simulink model "cooling_v3"  (R2022b)
settings: Solver=FixedStepDiscrete  StartTime=0.0  StopTime=10.0  FixedStep=0.005  RelTol=1e-3  EnableMultiTasking=on
PreLoadFcn:
  | try, model_open; catch, disp('Error occurred while executing model pre-load callback: model_open.m'); disp('Please assure that the MATLAB working directory is set to the model directory before opening.'); end
InitFcn:
  | try, model_open; catch, end
undefined symbols (not defined in the file): GCM, raptor_get_safe_string, raptor_xcp_function, sigbuilder_block
libraries: Raptor_lib x39, simulink x8, simulink_extras x1, dspswit3 x1, dspstat3 x1
CloseFcn:
  | try, model_close; catch, end
settings Model: Raptor_Target=GCM-1793-196-1503  Raptor_Calloc=NonVolatile (EEPROM)  RaptorUIDSize=4  RaptorBuildNum=0  Raptor_ecuaddr=11  RaptorFaultManager=Standard  RaptorFaultManagerAddXYCounts=1  Raptor_IsLiteMode=0  Creator=Ben  LastModifiedBy=jackh
settings SolverCC: AlgebraicLoopSolver=TrustRegion
settings DataIOCC: LimitDataPoints=on  SaveFormat=Array  SignalLoggingSaveFormat=ModelDataLogs  ReturnWorkspaceOutputs=off
settings OptimizationCC: DefaultParameterBehavior=Inlined  ExpressionDepthLimit=2147483647  InitFltsAndDblsToZero=on  LifeSpan=1  EfficientTunableParamExpr=on
settings DebuggingCC: SolverPrmCheckMsg=warning  InheritedTsInSrcMsg=none  ParameterPrecisionLossMsg=none  FcnCallInpInsideContextMsg=warning  UnconnectedInputMsg=warning  UnconnectedOutputMsg=warning  UnconnectedLineMsg=warning  StateNameClashWarn=warning  SFUnexpectedBacktrackingDiag=warning  SFNoUnconditionalDefaultTransitionDiag=warning  SFExecutionAtInitializationDiag=none  SFMachineParentedDataDiag=warning  ArithmeticOperatorsInVariantConditions=warning
settings HardwareCC: ProdBitPerPointer=32  ProdBitPerSizeT=32  ProdBitPerPtrDiffT=32  ProdLargestAtomicFloat=None  ProdWordSize=32  ProdHWDeviceType=Infineon->TriCore  TargetIntDivRoundTo=Zero  TargetEndianess=LittleEndian  ProdEqTarget=off
settings ModelReferenceCC: EnableRefExpFcnMdlSchedulingChecks=on  PropagateSignalLabelsOutOfModel=off
settings SFSimCC: SimUseLocalCustomCode=off  MATLABDynamicMemAlloc=off  CustomCodeUndefinedFunction=UseInterfaceOnly
settings RTWCC: Description=Raptor (tm)  SystemTargetFile=raptor.tlc  GenCodeOnly=on  MakeCommand=raptor_make_rtw  TemplateMakefile=raptor.tmf  RTWUseLocalCustomCode=off
settings CodeAppCC: IgnoreCustomStorageClasses=off  MaxIdLength=100  CustomSymbolStrType=$N$R$M  StateflowObjectComments=on  InternalIdentifier=Classic
settings STFCustomTargetCC: CodeReplacementLibrary=GCM196-specific  GenerateSampleERTMain=on  ModelReferenceCompliant=off  CombineOutputUpdateFcns=on  ERTCustomFileBanners=on  SupportContinuousTime=off  SupportNonInlinedSFcns=off  RemoveResetFunc=on  MATLABClassNameForMDSCustomization=Simulink.SoftwareTarget.ERTCustomization  SystemTargetFile=raptor.tlc
settings ERTTargetCC: CodeReplacementLibrary=GCM196-specific  MultiwordLength=2048  GenerateSampleERTMain=on  ModelReferenceCompliant=off  ParMdlRefBuildCompliant=off  CompOptLevelCompliant=off  ConcurrentExecutionCompliant=off  ModelStepFunctionPrototypeControlCompliant=off  CPPClassGenCompliant=off  UseToolchainInfoCompliant=off  ExtModeMexFile=noextcomm  InlinedParameterPlacement=NonHierarchical  ERTCustomFileTemplate=example_file_process.tlc  ConvertIfToSwitch=off  SuppressUnreachableDefaultCases=off
settings ConfigComp: CovMetricSettings=dw  CovSaveCumulativeToWorkspaceVar=on  CovSaveSingleToWorkspaceVar=on  CovExternalEMLEnable=off  CovSFcnEnable=off

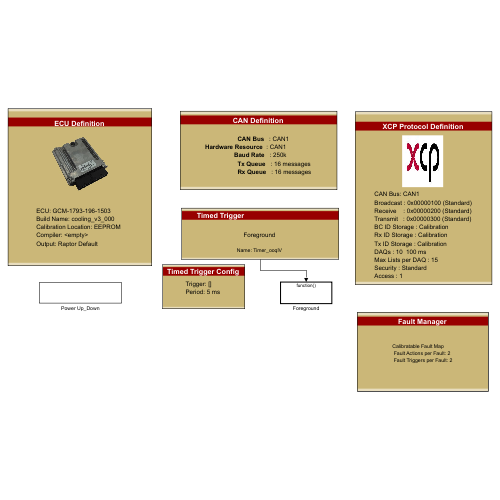
[thumbnail: Simulink's stored preview of the top-level diagram]
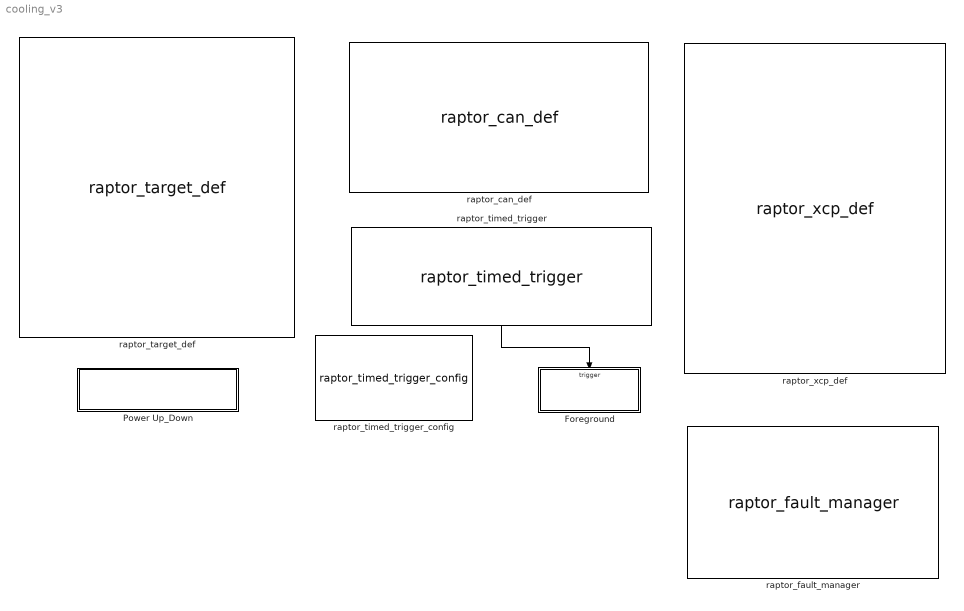
== system cooling_v3 ==
  Foreground : Subsystem  TreatAsAtomicUnit=on
      settings: RTWSystemCode=Nonreusable function
  Power Up_Down : Subsystem  mask{group='Diagnostics | Power Up_Down'}
  raptor_can_def : Raptor_lib/CAN/raptor_can_def  canBus='CAN1'  resourceValues=(None)|CAN1|CAN2  resource=CAN1  baudRateValues=250k  baudRate=250k  enable_baud_rate_config='RAPTOR MASK DEFAULT'  sim_func_name='RAPTOR MASK DEFAULT'  createButton=[]  txQueueSize=16  rxQueueSize=16
      settings: SourceProductName=Raptor
  raptor_fault_manager : Raptor_lib/Faults/raptor_fault_manager  button=0  managerTypeValues=Standard|OBD  managerType=Standard  cyclesToHeal=3  cyclesToClear=40  addXYCounts=1  calFaultMap=1  minFaultActions=2  minFaultTriggers=2  calAccessValues=4|3|2|1  calAccess=4  calFunction='System | FaultManager'  initMap=struct('managerType', 'Standard','actionMap', {{}},'triggerMap', {{}})  exportFilePath='C:\'  exportFileName='FaultMapExport_01.csv'
      settings: SourceProductName=Raptor
  raptor_target_def : Raptor_lib/Configuration/raptor_target_def  targetValues=BCM-5646-48-1404|DISP-VC128-1901|DISP-VC320L-1402|DISP-VC320-1204|DISP-VC800-1402|DISP-VC500-1904|DISP-VC700-2003|DISP-VC300R-2004|GCM-5634M-070-1459|GCM-5634M-070-1559|GCM-5634M-070-1562|ECM-1793-196-1503|GCM-1793-196-1503|GCM-5605B-048-1906|GCM-5605B-048-2104|GCM-5607B-80-1901|GCM-5607B-80-1903|GCM-5607B-80-2001|RCM-5743R-080-2005|RCM-5743R-080-2106|RCM-5743R-080-2203|UAS-5743R-047-2102|UAS-5743R-047-2107|GCM-5746R-048-1902|RCM-58NN-112-2007|RCM-58NN-112-2103|RCM-58NN-112-2202|HCM-5604-36-1303|HCM-5604-36-1702  target=GCM-1793-196-1503  simpack=0  simulator=0  heap=4*1024  stack=2*1024  fgndStack=3*1024  bgndStack=2*1024  idleStack=1024  intStack=1536  sdStack=1024  appStack=1024  ecuaddr=11  uds_server_addr_ext=0  uds_server_addr=hex2dec('600')  uds_client_addr=hex2dec('650')  callocValues=Constant (FLASH)|NonVolatile (EEPROM)  calloc=NonVolatile (EEPROM)  compilerValues=[]  compiler=<empty>  setFileName=0  exeName=[raptor_get_safe_string(bdroot) '_']  addBuildNum=1  minVerChars=3  extraOutput=0  buildLocationValues=Raptor Default|Model Directory|User Defined  buildLocation=Raptor Default  exeLocation=''  exeFileButton=0  a2lLocation=''  a2lFileButton=0  rpgLocation=''  rpgFileButton=0
      settings: SourceProductName=Raptor
  raptor_timed_trigger : Raptor_lib/Triggers/raptor_timed_trigger  triggerValues=Foreground|Foregroundx2|Foregroundx5|Foregroundx10|Foregroundx20|Background|Backgroundx2|Backgroundx5|Backgroundx10|Backgroundx20|Second|Minute|Task_1ms  trigger=Foreground  inherited=0  alwaysEnabled=1  triggerPriority=0  triggerName=ooqlV
      settings: SourceProductName=Raptor
  raptor_timed_trigger_config : Raptor_lib/Triggers/raptor_timed_trigger_config  triggerValues=[]  trigger=[]  period=5  CM2115newPeriod='RAPTOR MASK DEFAULT'
      settings: SourceProductName=Raptor
  raptor_xcp_def : Raptor_lib/Configuration/raptor_xcp_def  canBus='CAN1'  bcID=hex2dec('100')  bcID_TypeValues=Standard|Extended  bcID_Type=Standard  rxID=hex2dec('200')  rxID_TypeValues=Standard|Extended  rxID_Type=Standard  txID=hex2dec('300')  txID_TypeValues=Standard|Extended  txID_Type=Standard  daqRates=[10 100]  numODTs=15  genCANAPE=0  genVISION=0  securityValues=Standard|None|Custom User Defined  security=Standard  dllName=raptor_XCPSecurity.dll  accessValues=4|3|2|1  access=1  bcStorageValues=Constant (FLASH)|NonVolatile (EEPROM)|FixedNonVolatile (EEPROM)|Volatile (RAM)|Calibration  bcStorage=Calibration  txStorageValues=Constant (FLASH)|NonVolatile (EEPROM)|FixedNonVolatile (EEPROM)|Volatile (RAM)|Calibration  txStorage=Calibration  rxStorageValues=Constant (FLASH)|NonVolatile (EEPROM)|FixedNonVolatile (EEPROM)|Volatile (RAM)|Calibration  rxStorage=Calibration
      settings: SourceProductName=Raptor
  wires:
  raptor_timed_trigger/1 -> Foreground/Trigger

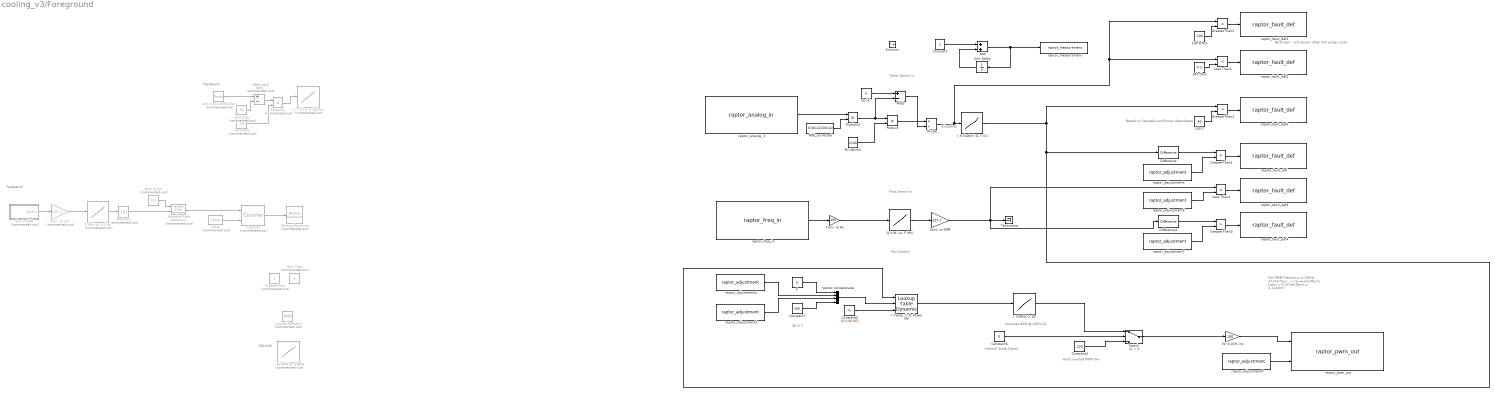
== system cooling_v3/Foreground ==
  note: Hold inverted PWM low
  note: Persistent - will remain after VCU power cycle
  note: Fan PWM Frequency is 24KHz
      | 5/(2*pi*tau) --> tau=Larm/Rarm
      | Larm = 0.137mH
      | Rarm = 4.114ohm
  note: Based on Cascadia and Emrax datasheets
  note: All in F
  note: Internal State Signal
  note: assumes 80W @ 100% DC
  note: CELCIUS
  note: Conv. to C
  note: KiloOHMS
  note: Testbench
  note: Testbench
  note: Temp Sensor In
  note: Fan Control
  note: Flow Sensor In
  function : TriggerPort  TriggerType=function-call  VariantControl=Variant
  100 C : Constant  Value=80
  100 Ohm : Constant  Value=0.1
  100 kOhm : Constant  Value=100
  ADC_corrected : Constant  Value=0.00122100122
  Add : Sum
  Add1 : Sum  Commented=on  Inputs=+-
  Add2 : Sum  Inputs=+-
  Clock : simulink_extras/Flip Flops/Clock  Commented=on  period=1
  Constant : Constant
  Constant1 : Constant  Commented=on  Value=32
  Constant2 : Constant  Commented=on  Value=5/9
  Constant4 : Constant  Value=100
  Constant5 : Constant  Value=[0;0;80;80]
  Constant6 : Constant  Value=0
  Constant7 : Constant  Value=300
  Conv. to GPM : Gain  Gain=227.1
  Conv. to Hz : Gain  Gain=100
  Conv. to L/H : Gain  Commented=on  Gain=1/227.1
  Counter : dspswit3/Counter  Commented=on  Direction=Up  CountEvent=Rising edge  CounterSize=User defined  MaxCount=255  InitialCount=0  Output=Count  HitValue=32  ResetInput=on  SamplesPerFrame=1  Ts=1  CntDtype=double  HitDtype=Logical
  Difference : simulink/Discrete/Difference  ICPrevInput=0.0  OutMin=[]  OutMax=[]  OutDataType=fixdt(1, 16)  OutScaling=2^-10  DoSatur=off
  Difference1 : simulink/Discrete/Difference  ICPrevInput=0.0  OutMin=[]  OutMax=[]  OutDataType=fixdt(1, 16)  OutScaling=2^-10  DoSatur=off
  Divide : Product  Inputs=*/
  Duty Cycle : Constant  Commented=on  Value=0.5
  F : Constant  Value=0
  F (Hz) vs. Q (L/H) : Lookup_n-D  Commented=on  NumberOfTableDimensions=1  BreakpointsForDimension1=[120;240;360;480;600;720]  Table=[16;32.5;49.3;65.5;82;90.2]  InternalRulePriority=Speed  RndMeth=Simplest
  GreaterThan : RelationalOperator  Commented=on  Operator=>  OutDataTypeStr=boolean  RndMeth=Simplest  InputSameDT=off
  GreaterThan{1..4} (4 alike) : RelationalOperator  Operator=>  OutDataTypeStr=boolean  RndMeth=Simplest  InputSameDT=off
  I: 0-80W O: DC : Lookup_n-D  NumberOfTableDimensions=1  BreakpointsForDimension1=[0;5;10;15;20;25;30;35;40;45;50;55;60;65;70;75;80]  Table=[100;93.75;87.5;81.25;75;68.75;62.5;56.25;50;43.75;37.5;31.25;25;18.75;12.5;6.25;0]  InternalRulePriority=Speed  RndMeth=Simplest
  "I: 65-300F O: 0-80W " : Lookup_n-D  Commented=on  NumberOfTableDimensions=1  BreakpointsForDimension1=[0;65;150;300]  Table=[0;0;80;80]  InternalRulePriority=Speed  RndMeth=Simplest
  I: R (kOhm) O: T (C) : Lookup_n-D  NumberOfTableDimensions=1  BreakpointsForDimension1=[0.583;0.6601;0.7487;0.8508;0.9688;1.106;1.265;1.452;1.67;1.928;2.232;2.593;3.025;3.541;4.163;4.914;5.827;6.942;8.311;10;12.1;14.71;17.99;22.13;27.39]  Table=[120;115;110;105;100;95;90;85;80;75;70;65;60;55;50;45;40;35;30;25;20;15;10;5;0]  InternalRulePriority=Speed  RndMeth=Simplest
  I: T (C) O: R (kOhm) : Lookup_n-D  Commented=on  NumberOfTableDimensions=1  BreakpointsForDimension1=[0;5;10;15;20;25;30;35;40;45;50;55;60;65;70;75;80;85;90;95;100;105;110;115;120]  Table=[27.39;22.13;17.99;14.71;12.1;10;8.311;6.942;5.827;4.914;4.163;3.541;3.025;2.593;2.232;1.928;1.67;1.452;1.265;1.106;0.9688;0.8508;0.7487;0.6601;0.583]  InternalRulePriority=Speed  RndMeth=Simplest
  I: Temp. () O: Power (W) : simulink/Lookup Tables/Lookup Table Dynamic  LookUpMeth=Interpolation-Use End Values  OutDataType=fixdt('double')  OutScaling=[]  OutputDataTypeScalingMode=Specify via dialog  OutDataTypeStr=double  DoSatur=off
  Less Than : RelationalOperator  Commented=on  Operator=<  OutDataTypeStr=boolean  RndMeth=Simplest  InputSameDT=off
  Less Than1 : RelationalOperator  Operator=<  OutDataTypeStr=boolean  RndMeth=Simplest  InputSameDT=off
  Less Than2 : RelationalOperator  Operator=<  OutDataTypeStr=boolean  RndMeth=Simplest  InputSameDT=off
  Logical Operator : Logic  Commented=on  AllPortsSameDT=off  OutDataTypeStr=boolean
  Moving Maximum : dspstat3/Moving Maximum  Commented=on  SpecifyWindowLength=on  WindowLength=4  SimulateUsing=Code generation
  PU (Ohms) : Constant  Value=2145
  Product : Product
  Product1 : Product  Commented=on
  Product2 : Product  Commented=on  Inputs=/
  Product3 : Product
  Q (L/H) vs. F (Hz) : Lookup_n-D  NumberOfTableDimensions=1  BreakpointsForDimension1=[16;32.5;49.3;65.5;82;90.2]  Table=[120;240;360;480;600;720]  ExtrapMethod=Clip  InternalRulePriority=Speed  RndMeth=Simplest
  Sim In GPM : Subsystem  Tag=STV Subsys  Commented=on  LoadFcn=sigbuilder_block('load');  StartFcn=sigbuilder_block('start');  StopFcn=sigbuilder_block('stop');  ClipboardFcn=sigbuilder_block('clipboard');  mask(Sigbuilder block){tuvar=[0:10]}
      mask help: Simulink:masks:SigbuilderBlock_MD
      mask init:
      | if ~strcmp(get_param(bdroot(gcbh),'SimulationStatus'),'stopped') tuvar = sigbuilder_block('maskInit'); end
      settings: CopyFcn=sigbuilder_block('copy');  DeleteFcn=sigbuilder_block('delete');  ModelCloseFcn=sigbuilder_block('modelClose');  PreSaveFcn=sigbuilder_block('preSave');  PauseFcn=sigbuilder_block('pause');  ContinueFcn=sigbuilder_block('continue');  NameChangeFcn=sigbuilder_block('namechange');  OpenFcn=sigbuilder_block('open',[437.6 199.2 550.4 400 ]);  CloseFcn=sigbuilder_block('close');
      mask Display: plot(0, 0, 100, 100,[2, 2, 32, 32, 2], [68, 8, 8, 68, 68],[32, 2], [38, 38], [32, 19, 2],[53, 60, 44], [32, 17, 17, 2],[16, 16, 31, 31]);txt = getActiveGroup(gcbh);text(2, 100, txt,'verticalAlignment', 'top');
  Sim In 65-130F/10min : simulink/Sources/Ramp  Commented=on  slope=0.1083  start=3  InitialOutput=0
  Switch : Switch  Criteria=u2 > Threshold  SaturateOnIntegerOverflow=off  InputSameDT=off
  Terminator : Terminator
  Unit Delay : UnitDelay  SampleTime=-1  HasFrameUpgradeWarning=on
  Variable Pulse Generator : VariablePulseGenerator  Commented=on  SampleTime=0.1
  Vector Concatenate : Concatenate  NumInputs=4
  Vs (V) : Constant  Value=5
  for 0.01% inc : Gain  Gain=100  OutDataTypeStr=Inherit: Inherit via back propagation
  raptor_adjustment2 : Raptor_lib/Data Storage/raptor_adjustment  paramName='LowerFanPoint'  nameSource=Parameter  initValue=65  dataType=double  storage=Calibration  calDispType=Number  calEnum={'False', 'True'}  calGain=1.0  calOffset=0.0  calMax=inf  calMin=-inf  calFormat='-1'  calUnit='F'  calHelp='Temp at 0W'  calAccess=1  calFunction=raptor_xcp_function(gcb)  calDispHeaders=off  calColHeaders={'Col1' 'Col2' 'Col3'}  calRowHeaders={'Row1' 'Row2' 'Row3'}
      settings: SourceProductName=Raptor
  raptor_adjustment3 : Raptor_lib/Data Storage/raptor_adjustment  paramName='UpperFanPoint'  nameSource=Parameter  initValue=150  dataType=double  storage=Calibration  calDispType=Number  calEnum={'False', 'True'}  calGain=1.0  calOffset=0.0  calMax=inf  calMin=-inf  calFormat='-1'  calUnit='F'  calHelp='Temp at 80W'  calAccess=1  calFunction=raptor_xcp_function(gcb)  calDispHeaders=off  calColHeaders={'Col1' 'Col2' 'Col3'}  calRowHeaders={'Row1' 'Row2' 'Row3'}
      settings: SourceProductName=Raptor
  raptor_adjustment4 : Raptor_lib/Data Storage/raptor_adjustment  paramName='FanFrequency'  nameSource=Parameter  initValue=2400000  dataType=uint32  storage=Calibration  calDispType=Number  calEnum={'False', 'True'}  calGain=100  calOffset=0.0  calMax=inf  calMin=-inf  calFormat='-1'  calUnit='Hz'  calHelp=''  calAccess=1  calFunction=raptor_xcp_function(gcb)  calDispHeaders=off  calColHeaders={'Col1' 'Col2' 'Col3'}  calRowHeaders={'Row1' 'Row2' 'Row3'}
      settings: SourceProductName=Raptor
  raptor_adjustment5 : Raptor_lib/Data Storage/raptor_adjustment  paramName='tempRateFault'  nameSource=Parameter  initValue=10  dataType=double  storage=Calibration  calDispType=Number  calEnum={'False', 'True'}  calGain=1.0  calOffset=0.0  calMax=inf  calMin=-inf  calFormat='-1'  calUnit='degC/sec'  calHelp=''  calAccess=1  calFunction=raptor_xcp_function(gcb)  calDispHeaders=off  calColHeaders={'Col1' 'Col2' 'Col3'}  calRowHeaders={'Row1' 'Row2' 'Row3'}
      settings: SourceProductName=Raptor
  raptor_adjustment6 : Raptor_lib/Data Storage/raptor_adjustment  paramName='lowFlowRateFault'  nameSource=Parameter  initValue=1  dataType=double  storage=Calibration  calDispType=Number  calEnum={'False', 'True'}  calGain=1.0  calOffset=0.0  calMax=inf  calMin=-inf  calFormat='-1'  calUnit='GPM'  calHelp=''  calAccess=1  calFunction=raptor_xcp_function(gcb)  calDispHeaders=off  calColHeaders={'Col1' 'Col2' 'Col3'}  calRowHeaders={'Row1' 'Row2' 'Row3'}
      settings: SourceProductName=Raptor
  raptor_adjustment7 : Raptor_lib/Data Storage/raptor_adjustment  paramName='eradicFlowRateFault'  nameSource=Parameter  initValue=10  dataType=double  storage=Calibration  calDispType=Number  calEnum={'False', 'True'}  calGain=1.0  calOffset=0.0  calMax=inf  calMin=-inf  calFormat='-1'  calUnit='deg/sec'  calHelp=''  calAccess=1  calFunction=raptor_xcp_function(gcb)  calDispHeaders=off  calColHeaders={'Col1' 'Col2' 'Col3'}  calRowHeaders={'Row1' 'Row2' 'Row3'}
      settings: SourceProductName=Raptor
  raptor_analog_in : Raptor_lib/Input & Output/raptor_analog_in  resourceValues=INPUT2|INPUT3|INPUT4|INPUT5|INPUT6|INPUT7|INPUT8|INPUT9|INPUT10|INPUT11|INPUT12|INPUT13|INPUT14|INPUT15|INPUT16|INPUT17|INPUT18|INPUT19|INPUT20|INPUT21|INPUT22|INPUT23|INPUT24|INPUT25|INPUT26|INPUT27|INPUT28|INPUT29|INPUT30|INPUT31|INPUT32|(None)  resource=INPUT21  pullUDValues=2.15k PU  pullUD=2.15k PU  rangeValues=0 - 5 V  range=0 - 5 V  filterrateValues=[]  filterrate='RAPTOR MASK DEFAULT'  resolutionValues=[]  resolution=[]
      settings: SourceProductName=Raptor
  raptor_fault_def : Raptor_lib/Faults/raptor_fault_def  faultName='eradicTemp'  persist=off  sticky=on  emisRelated=off  singleTrip=off  clearMethod=Standard  xLimit=25  yLimit=50  calEnable=on  addDisable=off  calAccess=1  calFunction='System | FaultManager'
      settings: SourceProductName=Raptor
  raptor_fault_def1 : Raptor_lib/Faults/raptor_fault_def  faultName='tempSenseOC'  persist=on  sticky=on  emisRelated=off  singleTrip=off  clearMethod=Standard  xLimit=25  yLimit=50  calEnable=on  addDisable=off  calAccess=1  calFunction='System | FaultManager'
      settings: SourceProductName=Raptor
  raptor_fault_def2 : Raptor_lib/Faults/raptor_fault_def  faultName='tempSenseSC'  persist=on  sticky=on  emisRelated=off  singleTrip=off  clearMethod=Standard  xLimit=25  yLimit=50  calEnable=on  addDisable=off  calAccess=1  calFunction='System | FaultManager'
      settings: SourceProductName=Raptor
  raptor_fault_def3 : Raptor_lib/Faults/raptor_fault_def  faultName='lowFlowRate'  persist=off  sticky=on  emisRelated=off  singleTrip=off  clearMethod=Standard  xLimit=25  yLimit=50  calEnable=on  addDisable=off  calAccess=1  calFunction='System | FaultManager'
      settings: SourceProductName=Raptor
  raptor_fault_def4 : Raptor_lib/Faults/raptor_fault_def  faultName='eradicFlow'  persist=off  sticky=on  emisRelated=off  singleTrip=off  clearMethod=Standard  xLimit=25  yLimit=50  calEnable=on  addDisable=off  calAccess=1  calFunction='System | FaultManager'
      settings: SourceProductName=Raptor
  raptor_fault_def5 : Raptor_lib/Faults/raptor_fault_def  faultName='tempHigh'  persist=off  sticky=on  emisRelated=off  singleTrip=off  clearMethod=Standard  xLimit=25  yLimit=50  calEnable=on  addDisable=off  calAccess=1  calFunction='System | FaultManager'
      settings: SourceProductName=Raptor
  raptor_freq_in : Raptor_lib/Input & Output/raptor_freq_in  resourceValues=INPUT41|INPUT42|INPUT43|INPUT44|INPUT45|(None)  resource=INPUT41  pullUDValues=[]  pullUD=[]  interfaceValues=[]  interface=[]  hasDuty=off  hasEdgeCount='RAPTOR MASK DEFAULT'
      settings: SourceProductName=Raptor
  raptor_measurement : Raptor_lib/Data Storage/raptor_measurement  paramName='Counter'  nameSource=Parameter  calDispType=Number  calEnum={'False', 'True'}  calGain=1.0  calOffset=0.0  calMax=inf  calMin=-inf  calFormat='-1'  calUnit=''  calHelp=''  calAccess=4  calFunction=raptor_xcp_function(gcb)  calVisible=on
      settings: SourceProductName=Raptor
  raptor_pwm_out : Raptor_lib/Input & Output/raptor_pwm_out  showEnable=0  resourceValues=OUTPUT1|OUTPUT2|OUTPUT3|OUTPUT4|OUTPUT5|OUTPUT6|OUTPUT7|OUTPUT8|OUTPUT9|OUTPUT10|OUTPUT11|OUTPUT12|(None)  resource=OUTPUT11  driverTypeValues=Low Side  driverType=Low Side
      settings: SourceProductName=Raptor
  wires:
  Constant/1 -> Add/1
  Add/1 -> raptor_measurement/1, Unit Delay/1
  Unit Delay/1 -> Add/2
  PU (Ohms)/1 -> Product/2
  Product/1 -> Divide/1
  Vs (V)/1 -> Add2/1
  Add2/1 -> Divide/2
  Divide/1 -> I: R (kOhm) O: T (C)/1, Less Than1/1, GreaterThan2/1
  Sim In 65-130F/10min/1 -> Add1/1
  Constant1/1 -> Add1/2
  Add1/1 -> Product1/1
  Product1/1 -> I: T (C) O: R (kOhm)/1
  Constant2/1 -> Product1/2
  I: R (kOhm) O: T (C)/1 -> GreaterThan4/1, I: Temp. () O: Power (W)/1, Difference/1
  Product2/1 -> Variable Pulse Generator/2
  Duty Cycle/1 -> Variable Pulse Generator/1
  Variable Pulse Generator/1 -> Counter/1
  Clock/1 -> Counter/2
  Counter/1 -> Moving Maximum/1
  Conv. to Hz/1 -> Q (L/H) vs. F (Hz)/1
  Q (L/H) vs. F (Hz)/1 -> Conv. to GPM/1
  F (Hz) vs. Q (L/H)/1 -> Product2/1
  Sim In GPM/1(Signal 1) -> Conv. to L/H/1
  Conv. to L/H/1 -> F (Hz) vs. Q (L/H)/1
  I: 0-80W O: DC/1 -> Switch/1
  raptor_freq_in/1 -> Conv. to Hz/1
  Constant4/1 -> Switch/3
  Switch/1 -> for 0.01% inc/1
  Constant5/1 -> I: Temp. () O: Power (W)/3
  F/1 -> Vector Concatenate/1
  Constant7/1 -> Vector Concatenate/4
  Vector Concatenate/1 -> I: Temp. () O: Power (W)/2
  raptor_adjustment3/1 -> Vector Concatenate/3
  raptor_adjustment2/1 -> Vector Concatenate/2
  I: Temp. () O: Power (W)/1 -> I: 0-80W O: DC/1
  Conv. to GPM/1 -> Difference1/1, Less Than2/1, Terminator/1
  Constant6/1 -> Switch/2
  raptor_adjustment4/1 -> raptor_pwm_out/2
  for 0.01% inc/1 -> raptor_pwm_out/1
  Difference/1 -> GreaterThan1/1
  GreaterThan1/1 -> raptor_fault_def/1
  raptor_adjustment5/1 -> GreaterThan1/2
  GreaterThan2/1 -> raptor_fault_def1/1
  100 kOhm/1 -> GreaterThan2/2
  Less Than1/1 -> raptor_fault_def2/1
  100 Ohm/1 -> Less Than1/2
  raptor_adjustment6/1 -> Less Than2/2
  Less Than2/1 -> raptor_fault_def3/1
  GreaterThan3/1 -> raptor_fault_def4/1
  raptor_adjustment7/1 -> GreaterThan3/2
  Difference1/1 -> GreaterThan3/1
  GreaterThan4/1 -> raptor_fault_def5/1
  100 C/1 -> GreaterThan4/2
  raptor_analog_in/1 -> Product3/1
  ADC_corrected/1 -> Product3/2
  Product3/1 -> Add2/2, Product/1

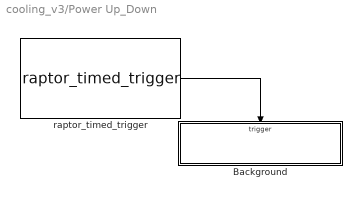
== system cooling_v3/Power Up_Down ==
  Background : Subsystem
  raptor_timed_trigger : Raptor_lib/Triggers/raptor_timed_trigger  triggerValues=Foreground|Foregroundx2|Foregroundx5|Foregroundx10|Foregroundx20|Background|Backgroundx2|Backgroundx5|Backgroundx10|Backgroundx20|Second|Minute  trigger=Background  inherited=0  alwaysEnabled=1  triggerPriority=50  triggerName=BGND_G6Wyo
      settings: SourceProductName=Raptor
  wires:
  raptor_timed_trigger/1 -> Background/Trigger

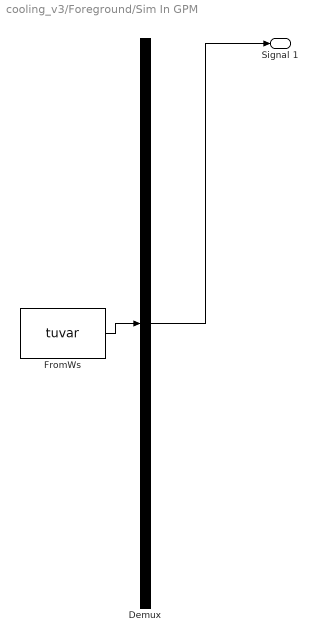
== system cooling_v3/Foreground/Sim In GPM ==
  Demux : Demux  Tag=STV Demux  Outputs=1
      settings: DisplayOption=none
  FromWs : FromWorkspace  Tag=STV FromWs  VariableName=tuvar
      SigBuilderData=|
      | common.afterFinalStr = 'Extrapolate'
      | common.sampleTime = 0
      | dataSet.timeRange = [0 10]
      | dataSet.name = 'Group 1'
      | sbobj.Groups.Name = 'Group 1'
      | sbobj.Groups.Signals.Name = 'Signal 1'
      | sbobj.Groups.Signals.XData = [0 4 4 6 6 10]
      | sbobj.Groups.Signals.YData = [0 0 1 1 0 0]
  Signal 1 : Outport  Tag=STV Outport
  wires:
  Demux/1 -> Signal 1/1
  FromWs/1 -> Demux/1

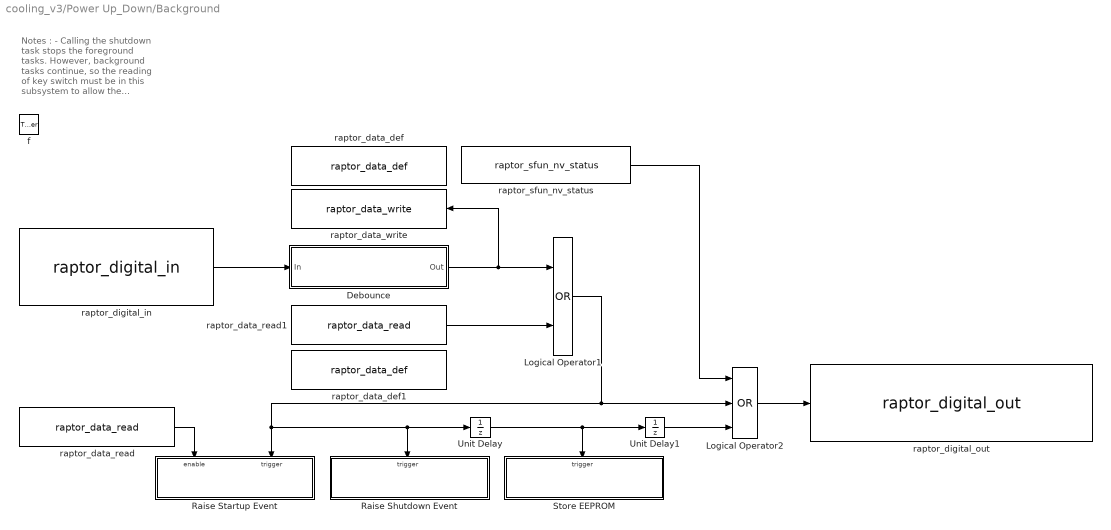
== system cooling_v3/Power Up_Down/Background ==
  note: Notes :
      | - Calling the shutdown task stops the foreground tasks. However, background tasks continue, so the reading of key switch must be in this subsystem to allow the module
      | to resume operation (by calling the startup task) if keyswitch is turned back on before the module actually turns off.
      | - The Startup Event is automatically called when the module is powered on after being completely off. The FgndTasksStopped data store prevents the Startup Event from being called twice in this scenario.
  f : TriggerPort  TriggerType=function-call  VariantControl=Variant  ZeroCross=off
  Debounce : Subsystem
  Logical Operator1 : Logic  Operator=OR  OutDataTypeStr=boolean
  Logical Operator2 : Logic  Operator=OR  Inputs=3  OutDataTypeStr=boolean
  Raise Shutdown Event : Subsystem  TreatAsAtomicUnit=on
  Raise Startup Event : Subsystem  TreatAsAtomicUnit=on
  Store EEPROM : Subsystem  TreatAsAtomicUnit=on
  Unit Delay : UnitDelay  SampleTime=-1  HasFrameUpgradeWarning=on
  Unit Delay1 : UnitDelay  SampleTime=-1  HasFrameUpgradeWarning=on
  raptor_data_def : Raptor_lib/Data Storage/raptor_data_def  dataName='KeySw_Bgnd'  initValue=0  dataType=boolean  storage=Volatile (RAM)  calVisible=on  calType=Measurement  calDispType=Number  calEnum={'False', 'True'}  calGain=1.0  calOffset=0  calMin=-Inf  calMax=Inf  calFormat='-1'  calUnit='Bool'  calHelp='Key switch reading from background task'  calAccess=1  calFunction=group  calDispHeaders=off  calColHeaders={'Col1' 'Col2' 'Col3'}  calRowHeaders={'Row1' 'Row2' 'Row3'}
      settings: SourceProductName=Raptor
  raptor_data_def1 : Raptor_lib/Data Storage/raptor_data_def  dataName='KeepModuleOn'  initValue=0  dataType=boolean  storage=Volatile (RAM)  calVisible=on  calType=Measurement  calDispType=Number  calEnum={'False', 'True'}  calGain=1.0  calOffset=0  calMin=-Inf  calMax=Inf  calFormat='-1'  calUnit='Bool'  calHelp='Boolean indicating module to be kept on'  calAccess=1  calFunction=group  calDispHeaders=off  calColHeaders={'Col1' 'Col2' 'Col3'}  calRowHeaders={'Row1' 'Row2' 'Row3'}
      settings: SourceProductName=Raptor
  raptor_data_read : Raptor_lib/Data Storage/raptor_data_read  dataName='FgndTasksStopped'  dataShape=Scalar  idxSource=Input  idxRow=1  idxCol=1
      settings: SourceProductName=Raptor
  raptor_data_read1 : Raptor_lib/Data Storage/raptor_data_read  dataName='KeepModuleOn'  dataShape=Scalar  idxSource=Input  idxRow=1  idxCol=1
      settings: SourceProductName=Raptor
  raptor_data_write : Raptor_lib/Data Storage/raptor_data_write  dataName='KeySw_Bgnd'  dataShape=Scalar  idxSource=Input Port  idxRow=1  idxCol=1
      settings: SourceProductName=Raptor
  raptor_digital_in : Raptor_lib/Input & Output/raptor_digital_in  resourceValues=(None)|WAKE_INPUT1|INPUT33|INPUT34|INPUT35|INPUT36|INPUT37|INPUT38|INPUT39|INPUT40  resource=WAKE_INPUT1  pullUDValues=2.9k PD  pullUD=2.9k PD  upperThres=1.980  lowerThres=1.320
      settings: SourceProductName=Raptor
  raptor_digital_out : Raptor_lib/Input & Output/raptor_digital_out  resourceValues=OUTPUT9|OUTPUT21|OUTPUT22|OUTPUT23|OUTPUT24|(None)|OUTPUT1|OUTPUT2|OUTPUT3|OUTPUT4|OUTPUT5|OUTPUT6|OUTPUT7|OUTPUT8|OUTPUT10|OUTPUT11|OUTPUT25|OUTPUT26|OUTPUT27|OUTPUT28|OUTPUT29|OUTPUT30|OUTPUT31|OUTPUT32|OUTPUT33|OUTPUT34|OUTPUT35|OUTPUT36|OUTPUT37|OUTPUT38|OUTPUT39|OUTPUT40|OUTPUT41|OUTPUT42|OUTPUT43|OUTPUT44|OUTPUT45|OUTPUT46|OUTPUT47|OUTPUT48|POWER_HOLD  resource=POWER_HOLD  driverTypeValues=(None)  driverType=(None)
      settings: SourceProductName=Raptor
  raptor_sfun_nv_status : Raptor_lib/Data Storage/raptor_sfun_nv_status  showStatus=Store In Progess
      settings: SourceProductName=Raptor
  wires:
  raptor_data_read/1 -> Raise Startup Event/Enable
  raptor_digital_in/1 -> Debounce/1(In)
  Logical Operator2/1 -> raptor_digital_out/1
  Unit Delay/1 -> Store EEPROM/Trigger, Unit Delay1/1
  Logical Operator1/1 -> Logical Operator2/2, Raise Startup Event/Trigger, Raise Shutdown Event/Trigger, Unit Delay/1
  Unit Delay1/1 -> Logical Operator2/3
  raptor_sfun_nv_status/1 -> Logical Operator2/1
  raptor_data_read1/1 -> Logical Operator1/2
  Debounce/1(Out) -> raptor_data_write/1, Logical Operator1/1

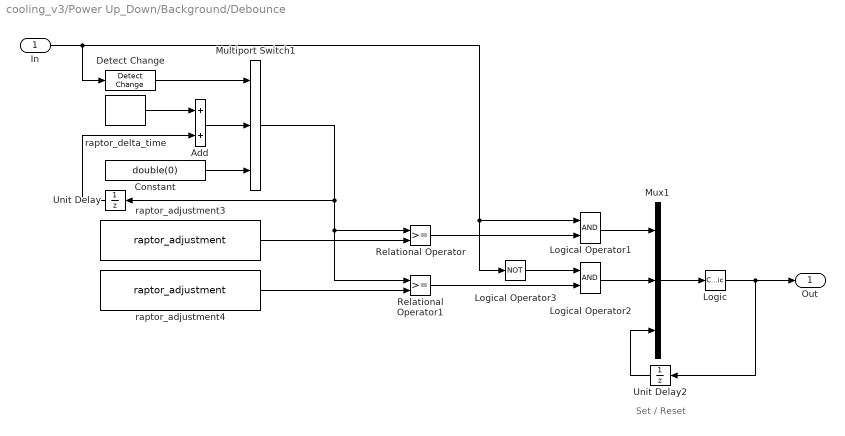
== system cooling_v3/Power Up_Down/Background/Debounce ==
  note: Set / Reset
  In : Inport
  Add : Sum
  Constant : Constant  Value=double(0)
  Detect Change : simulink/Logic and Bit Operations/Detect Change  vinit=0  OutDataTypeStr=boolean
  Logic : CombinatorialLogic  TruthTable=[0;1;0;0;1;1;0;0]
  Logical Operator1 : Logic  AllPortsSameDT=off  OutDataTypeStr=boolean
  Logical Operator2 : Logic  AllPortsSameDT=off  OutDataTypeStr=boolean
  Logical Operator3 : Logic  Operator=NOT  Inputs=1  AllPortsSameDT=off  OutDataTypeStr=boolean
  Multiport Switch1 : MultiPortSwitch  DataPortOrder=Zero-based contiguous  Inputs=2  zeroidx=on  SaturateOnIntegerOverflow=off  InputSameDT=off
  Mux1 : Mux  Inputs=3
  Relational Operator : RelationalOperator  OutDataTypeStr=boolean  InputSameDT=off
  Relational Operator1 : RelationalOperator  OutDataTypeStr=boolean  InputSameDT=off
  Unit Delay : UnitDelay  SampleTime=-1  HasFrameUpgradeWarning=on
  Unit Delay2 : UnitDelay  InitialCondition=1  SampleTime=-1  HasFrameUpgradeWarning=on
  raptor_adjustment3 : Raptor_lib/Data Storage/raptor_adjustment  paramName='KeySwHiTimeThr'  nameSource=Parameter  initValue=0.2  dataType=double  storage=Calibration  calDispType=Number  calEnum={'Active Low', 'Active High'}  calGain=1  calOffset=0  calMax=inf  calMin=-inf  calFormat='-1'  calUnit='sec'  calHelp='State high time threshold'  calAccess=1  calFunction=group  calDispHeaders=off  calColHeaders={'Col1' 'Col2' 'Col3'}  calRowHeaders={'Row1' 'Row2' 'Row3'}
      settings: SourceProductName=Raptor
  raptor_adjustment4 : Raptor_lib/Data Storage/raptor_adjustment  paramName='KeySwLoTimeThr'  nameSource=Parameter  initValue=0.2  dataType=double  storage=Calibration  calDispType=Number  calEnum={'Active Low', 'Active High'}  calGain=1  calOffset=0  calMax=inf  calMin=-inf  calFormat='-1'  calUnit='sec'  calHelp='State low time threshold'  calAccess=1  calFunction=group  calDispHeaders=off  calColHeaders={'Col1' 'Col2' 'Col3'}  calRowHeaders={'Row1' 'Row2' 'Row3'}
      settings: SourceProductName=Raptor
  raptor_delta_time : Raptor_lib/Triggers/raptor_delta_time  unit=seconds
      settings: SourceProductName=Raptor
  Out : Outport  VectorParamsAs1DForOutWhenUnconnected=off
  wires:
  Detect Change/1 -> Multiport Switch1/1
  Logical Operator3/1 -> Logical Operator2/1
  Relational Operator/1 -> Logical Operator1/2
  Logical Operator2/1 -> Mux1/2
  Logical Operator1/1 -> Mux1/1
  Mux1/1 -> Logic/1
  Unit Delay2/1 -> Mux1/3
  In/1 -> Detect Change/1, Logical Operator1/1, Logical Operator3/1
  Multiport Switch1/1 -> Unit Delay/1, Relational Operator/1, Relational Operator1/1
  Add/1 -> Multiport Switch1/2
  Constant/1 -> Multiport Switch1/3
  Relational Operator1/1 -> Logical Operator2/2
  Logic/1 -> Unit Delay2/1, Out/1
  Unit Delay/1 -> Add/2
  raptor_delta_time/1 -> Add/1
  raptor_adjustment4/1 -> Relational Operator1/2
  raptor_adjustment3/1 -> Relational Operator/2

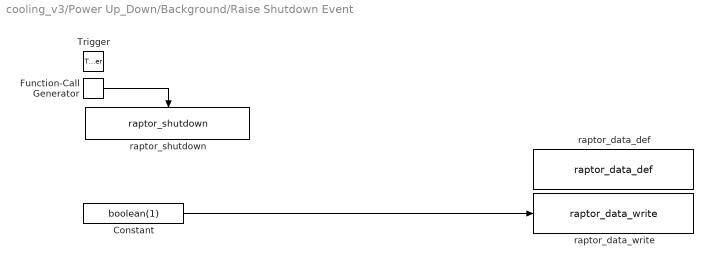
== system cooling_v3/Power Up_Down/Background/Raise Shutdown Event ==
  Trigger : TriggerPort  TriggerType=falling  VariantControl=Variant
  Constant : Constant  Value=boolean(1)
  Function-Call Generator : simulink/Ports & Subsystems/Function-Call Generator  sample_time=-1  numberOfIterations=1  DisallowWideOutput=off
  raptor_data_def : Raptor_lib/Data Storage/raptor_data_def  dataName='FgndTasksStopped'  initValue=0  dataType=boolean  storage=Volatile (RAM)  calVisible=on  calType=Measurement  calDispType=Number  calEnum={'False', 'True'}  calGain=1.0  calOffset=0  calMin=-Inf  calMax=Inf  calFormat='-1'  calUnit='Bool'  calHelp='Boolean indicating foreground tasks stopped'  calAccess=1  calFunction=group  calDispHeaders=off  calColHeaders={'Col1' 'Col2' 'Col3'}  calRowHeaders={'Row1' 'Row2' 'Row3'}
      settings: SourceProductName=Raptor
  raptor_data_write : Raptor_lib/Data Storage/raptor_data_write  dataName='FgndTasksStopped'  dataShape=Scalar  idxSource=Input Port  idxRow=1  idxCol=1
      settings: SourceProductName=Raptor
  raptor_shutdown : Raptor_lib/Triggers/raptor_shutdown  null=0
      settings: SourceProductName=Raptor
  wires:
  Constant/1 -> raptor_data_write/1
  Function-Call Generator/1 -> raptor_shutdown/Trigger

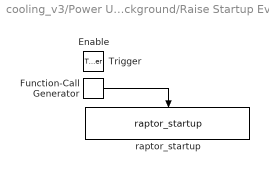
== system cooling_v3/Power Up_Down/Background/Raise Startup Event ==
  Enable : EnablePort
  Trigger : TriggerPort  VariantControl=Variant
  Function-Call Generator : simulink/Ports & Subsystems/Function-Call Generator  sample_time=-1  numberOfIterations=1  DisallowWideOutput=off
  raptor_startup : Raptor_lib/Triggers/raptor_startup  null=0
      settings: SourceProductName=Raptor
  wires:
  Function-Call Generator/1 -> raptor_startup/Trigger

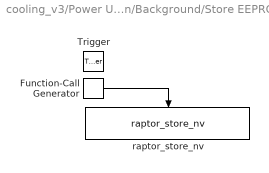
== system cooling_v3/Power Up_Down/Background/Store EEPROM ==
  Trigger : TriggerPort  TriggerType=falling  VariantControl=Variant
  Function-Call Generator : simulink/Ports & Subsystems/Function-Call Generator  sample_time=-1  numberOfIterations=1  DisallowWideOutput=off
  raptor_store_nv : Raptor_lib/Data Storage/raptor_store_nv  null=0
      settings: SourceProductName=Raptor
  wires:
  Function-Call Generator/1 -> raptor_store_nv/Trigger
